simulink model "rdr_model"  (R2015a)
settings: configuration reference "config_cosim" (kept outside this file)
undefined symbols (not defined in the file): dsm_pcs_tgt, pos_rdr_ini
settings Model: CovModelRefEnable=off  Creator=ericli  LastModifiedBy=ericli
settings ConfigSetRef: SourceLocation=Base Workspace

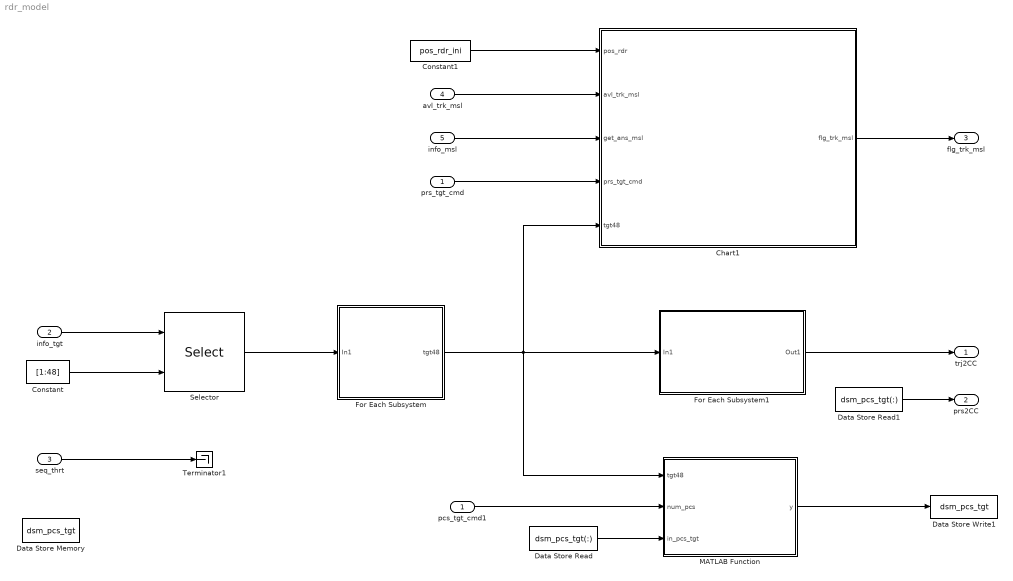
== system rdr_model ==
  prs_tgt_cmd : Inport  Description=指控发控给的目指标识及对应航迹编号
  info_tgt : Inport  Port=2  OutDataTypeStr=Bus: bus_new_tgt  PortDimensions=100  BusOutputAsStruct=on
  seq_thrt : Inport  Port=3  OutDataTypeStr=Bus: BusObject_threat_CC2rdr  PortDimensions=48  BusOutputAsStruct=on
  avl_trk_msl : Inport  Port=4
  info_msl : Inport  Port=5
  Chart1 : Stateflow chart  TreatAsAtomicUnit=on
  Constant : Constant  Value=[1:48]
  Constant1 : Constant  Value=pos_rdr_ini
  Data Store Memory : DataStoreMemory  DataStoreName=dsm_pcs_tgt  ReadBeforeWriteMsg=warning  WriteAfterWriteMsg=warning  WriteAfterReadMsg=warning  InitialValue=one_pcs_tgt  OutDataTypeStr=Bus: bus_pcs_tgt  Dimensions=8
  Data Store Read : DataStoreRead  DataStoreName=dsm_pcs_tgt  DataStoreElements=dsm_pcs_tgt(:)
  Data Store Read1 : DataStoreRead  DataStoreName=dsm_pcs_tgt  DataStoreElements=dsm_pcs_tgt(:)
  Data Store Write1 : DataStoreWrite  DataStoreName=dsm_pcs_tgt
  For Each Subsystem : Subsystem  TreatAsAtomicUnit=on
  For Each Subsystem1 : Subsystem  TreatAsAtomicUnit=on
  MATLAB Function : MATLAB Function  TreatAsAtomicUnit=on
  Selector : Selector  InputPortWidth=100  IndexOptions=Index vector (port)  Indices=[1 3]
  Terminator1 : Terminator
  pcs_tgt_cmd1 : InportShadow  Description=指控发控给的目指标识及对应航迹编号
  trj2CC : Outport  OutDataTypeStr=Bus: BusObject_tgt_rdr2CC  PortDimensions=48  BusOutputAsStruct=on
  prs2CC : Outport  Port=2  OutDataTypeStr=Bus: bus_pcs_tgt  PortDimensions=8  BusOutputAsStruct=on
  flg_trk_msl : Outport  Port=3
  wires:
  Constant1/1 -> Chart1/1(pos_rdr)
  Selector/1 -> For Each Subsystem/1(In1)
  info_tgt/1 -> Selector/1
  Constant/1 -> Selector/2
  For Each Subsystem1/1(Out1) -> trj2CC/1
  Data Store Read1/1 -> prs2CC/1
  avl_trk_msl/1 -> Chart1/2(avl_trk_msl)
  prs_tgt_cmd/1 -> Chart1/4(prs_tgt_cmd)
  seq_thrt/1 -> Terminator1/1
  pcs_tgt_cmd1/1 -> MATLAB Function/2(num_pcs)
  Data Store Read/1 -> MATLAB Function/3(in_pcs_tgt)
  MATLAB Function/1(y) -> Data Store Write1/1
  info_msl/1 -> Chart1/3(get_ans_msl)
  Chart1/1(flg_trk_msl) -> flg_trk_msl/1
  For Each Subsystem/1(tgt48) -> Chart1/5(tgt48), For Each Subsystem1/1(In1), MATLAB Function/1(tgt48)

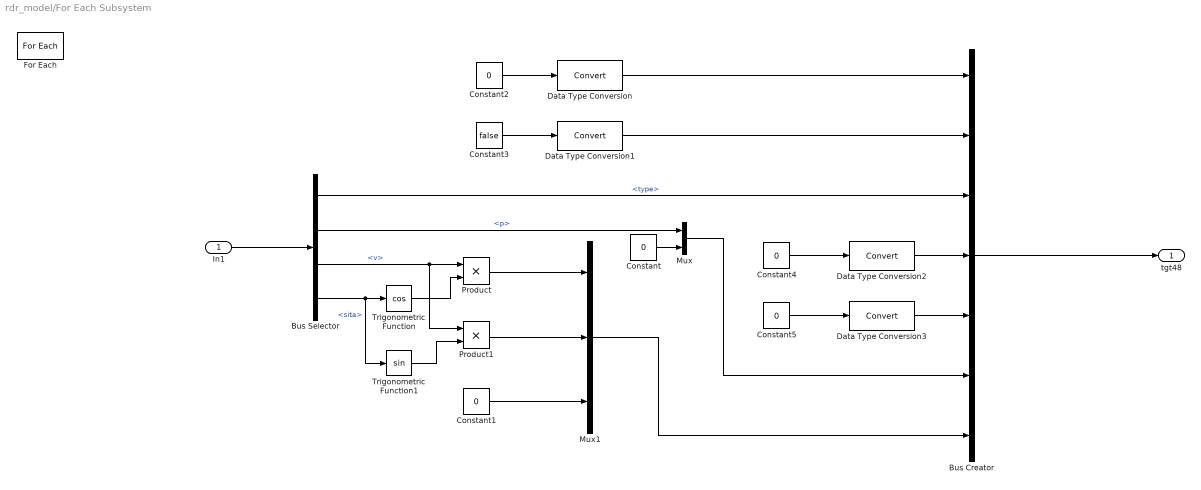
== system rdr_model/For Each Subsystem ==
  In1 : Inport  Partition=on  PartitionDimension=1  PartitionWidth=1
  Bus Creator : BusCreator  Inputs=7  OutDataTypeStr=Bus: bus_trj_tgt  NonVirtualBus=on
      settings: InheritFromInputs=off
  Bus Selector : BusSelector  OutputSignals=type,p,v,sita
  Constant{,1..2,4..5} (5 alike) : Constant  Value=0
  Constant3 : Constant  Value=false
  Data Type Conversion{,1..3} (4 alike) : DataTypeConversion
  For Each : ForEach  DisableCoverage=on  IndexMode=One-based
  Mux : Mux  Inputs=2
  Mux1 : Mux  Inputs=3
  Product : Product
  Product1 : Product
  Trigonometric Function : Trigonometry  Operator=cos
  Trigonometric Function1 : Trigonometry
  tgt48 : Outport  ConcatenationDimension=1
  wires:
  Bus Selector/4 -> Trigonometric Function1/1, Trigonometric Function/1  "<sita>"
  In1/1 -> Bus Selector/1
  Bus Selector/2 -> Mux/1  "<p>"
  Constant/1 -> Mux/2
  Trigonometric Function/1 -> Product/2
  Bus Selector/3 -> Product1/1, Product/1  "<v>"
  Trigonometric Function1/1 -> Product1/2
  Product/1 -> Mux1/1
  Product1/1 -> Mux1/2
  Constant1/1 -> Mux1/3
  Bus Creator/1 -> tgt48/1
  Constant2/1 -> Data Type Conversion/1
  Data Type Conversion/1 -> Bus Creator/1
  Constant3/1 -> Data Type Conversion1/1
  Bus Selector/1 -> Bus Creator/3  "<type>"
  Constant4/1 -> Data Type Conversion2/1
  Constant5/1 -> Data Type Conversion3/1
  Mux/1 -> Bus Creator/6
  Mux1/1 -> Bus Creator/7
  Data Type Conversion1/1 -> Bus Creator/2
  Data Type Conversion2/1 -> Bus Creator/4
  Data Type Conversion3/1 -> Bus Creator/5

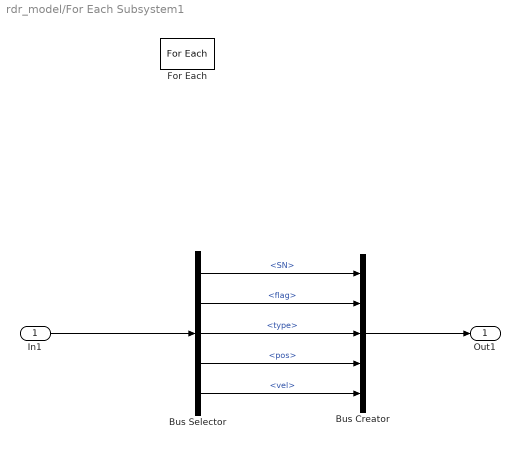
== system rdr_model/For Each Subsystem1 ==
  In1 : Inport  Partition=on  PartitionDimension=1  PartitionWidth=1
  Bus Creator : BusCreator  Inputs=5  OutDataTypeStr=Bus: BusObject_tgt_rdr2CC  NonVirtualBus=on
      settings: InheritFromInputs=off
  Bus Selector : BusSelector  OutputSignals=SN,flag,type,pos,vel
  For Each : ForEach  DisableCoverage=on  IndexMode=One-based
  Out1 : Outport  ConcatenationDimension=1
  wires:
  In1/1 -> Bus Selector/1
  Bus Selector/1 -> Bus Creator/1  "<SN>"
  Bus Selector/2 -> Bus Creator/2  "<flag>"
  Bus Selector/3 -> Bus Creator/3  "<type>"
  Bus Selector/4 -> Bus Creator/4  "<pos>"
  Bus Selector/5 -> Bus Creator/5  "<vel>"
  Bus Creator/1 -> Out1/1

== stateflow chart rdr_model/Chart1 ==
  state ini
    (default) -> (junction 28) : {
        | lat_rdr = pos_rdr(1);
        | lon_rdr = pos_rdr(2);
        | alt_rdr = pos_rdr(3);
        | flg_rdr =  true;
        | }
  state work
    state TGT [parallel]
      settings: executionOrder=1
    state MSL [parallel]
      settings: executionOrder=2  description=2.5.4
      state standby
      state capture
        state ANS1 [parallel]
          settings: executionOrder=1
          state no
            en:
            flg_ans_msl = false;
          state yes
            en:
            flg_ans_msl = true;
          (default) -> no
          yes -> no : [~get_ans_msl]
          no -> yes : [get_ans_msl]
        state CPT [parallel]
          settings: executionOrder=2
          state no_cpt
            en:
            flg_trk_msl = false;
          state yes_cpt
            en:
            flg_trk_msl = true;
          (default) -> no_cpt
          yes_cpt -> no_cpt : [~flg_ans_msl]
          no_cpt -> yes_cpt : [flg_ans_msl]
      (default) -> standby
      standby -> capture : [avl_trk_msl]
  (default) -> ini
  ini -> work : [flg_rdr]
  data: pos_rdr input; alt_rdr local; lon_rdr local; lat_rdr local; flg_rdr local; avl_trk_msl input boolean; flg_trk_msl output; get_ans_msl input; flg_ans_msl local; prs_tgt_cmd input size=8; tgt48 input size=48

== matlab function rdr_model/MATLAB Function ==
  data: tgt48 input Bus: bus_trj_tgt; y output Bus: bus_pcs_tgt; num_pcs input; in_pcs_tgt input Bus: bus_pcs_tgt size=8
function y = fcn(tgt48,num_pcs,in_pcs_tgt)
%#codegen

% if num_pcs<1
%     error('input 2 must be a positive integer number');
% end
y = in_pcs_tgt;
len = length(num_pcs);
for i=1:len
    if num_pcs(i)>0
        y(i).flag = FlagPcs.tracked;
        y(i).data = tgt48(num_pcs(i));
    end
    
end
